simulink model "sampleModel1592"  (R2023a)
settings: Solver=VariableStepAuto  StartTime=0.0  StopTime=10.0  RelTol=1e-3
libraries: hdlsllib x2, simulink x1
settings Model: Creator=user1  LastModifiedBy=user1

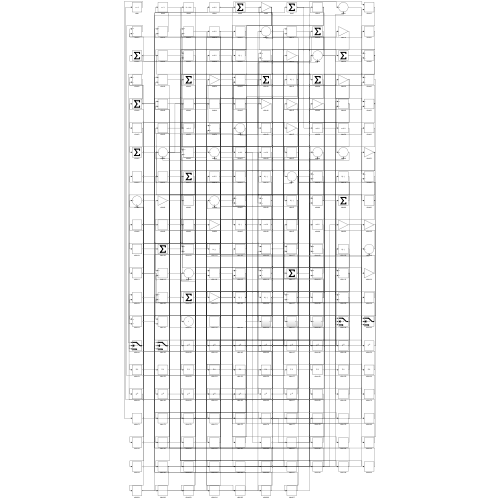
[thumbnail: Simulink's stored preview of the top-level diagram]
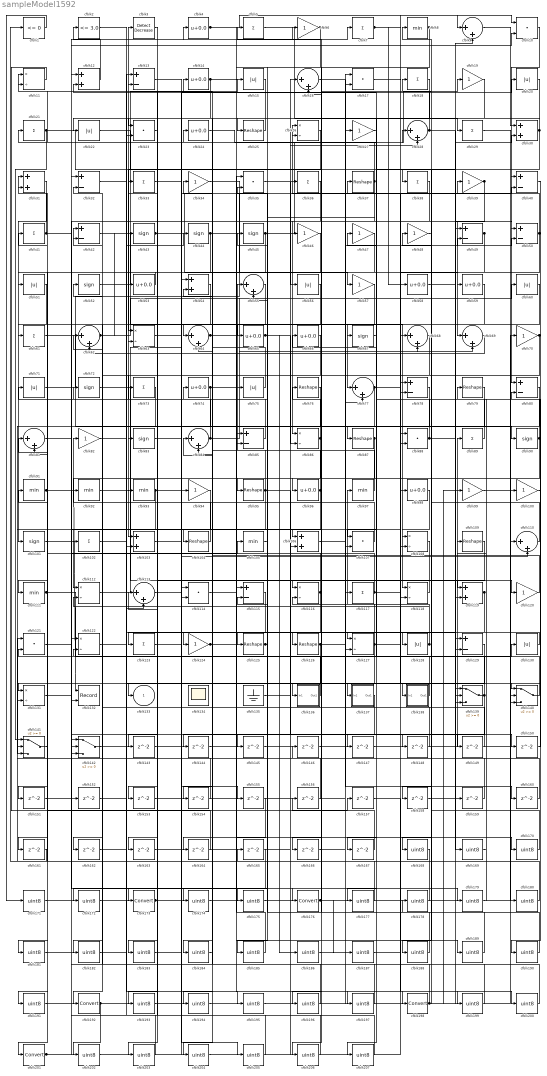
== system sampleModel1592 ==
  cfblk1 : hdlsllib/Logic and Bit Operations/Compare To Zero  relop=<=  OutDataTypeStr=boolean
  cfblk{10,17,23,35,88,107,114,121} (8 alike) : DotProduct  OutDataTypeStr=Inherit: Inherit via internal rule
  cfblk{6,19,27,34,39,46..48,57,70,82,94,99..100,120,124} (16 alike) : Gain
  cfblk{43..45,52,67,72,83,90,101} (9 alike) : Signum
  cfblk{5,7,18,21,29,33,36,38,41,61,73,89,102,117,123} (15 alike) : Sum  Inputs=+
  cfblk{12,30..31,54,103,106,119} (7 alike) : Sum
  cfblk{25,37,76,79,87,95,104,109,125..126} (10 alike) : Reshape
  cfblk{8,91..93,97,105,111} (7 alike) : MinMax
  cfblk{11,26,63,86,108,112,116,118,122,127,131} (11 alike) : Product  Inputs=*/  RndMeth=Zero  SaturateOnIntegerOverflow=on
  cfblk{9,16,28,55,62,64,68..69,77,81,84,110,113} (13 alike) : Sum  Inputs=|++
  cfblk{13,32,40,42,49..50,78,80,85,115,129} (11 alike) : Sum  Inputs=+-
  cfblk{15,20,22,51,56,60,71,75,128,130} (10 alike) : Abs  SaturateOnIntegerOverflow=off
  cfblk132 : Record  FileSettingsInternal="{\"entries\":[{\"content\":{\"excelSettings\":{\"content\":{},\"type\":\"Streamout.ExcelSettings\"}},\"type\":\"Streamout.FileSettingStorage\",\"uuid\":\"\"}],\"packageUris\":[\"http:\\/\\/schema.mathworks.com\\/mf0\\/streamout_blocks\\/R2020a\"],\"version\":\"1.0\"}"  Layout=[1 1]  SignalsInternal="{\"entries\":[{\"content\":{\"signals\":[{\"content\":{\"blockPath\":[],\"dimensions\":[1],\"domain\":\"\",\"lineColor\":\"#a2142f\",\"plots\":[1],\"port\":1,\"signalID\":2175,\"signalName\":\"XY Graph:1\"},\"type\":\"RecordBlkView.Signal\",\"uuid\":\"\"},{\"content\":{\"blockPath\":[],\"dimensions\":[1],\"domain\":\"\",\"lineColor\":\"#139fff\",\"plots\":[1],\"port\":2,\"signalID\":2178,\"signalName\":\"XY Graph:2\"},\"type\":\"RecordBlkView.Signal\",\"uuid\":\"\"}]},\"type\":\"RecordBlkView.InputSignals\",\"uuid\":\"\"}],\"packageUris\":[\"http:\\/\\/schema.mathworks.com\\/mf0\\/streamout_blocks\\/R2020a\"],\"version\":\"1.0\"}"  VisualizationBindings="{\"xyplotplugin\":{\"info\":[{\"series\":[{\"bindingParametersList\":[{\"parameter\":\"X-Axis\",\"signalID\":2175,\"signalName\":\"XY Graph:1\"},{\"parameter\":\"Y-Axis\",\"signalID\":2178,\"signalName\":\"XY Graph:2\"}],\"seriesID\":40184}],\"subplotID\":1}]}}"  CompatibilityTag=XY  st=-1
  cfblk134 : Scope
      settings: Floating=on
  cfblk135 : Ground
  cfblk136 : Subsystem
      settings: LibrarySourceBlock=|
      | hdlsllib/Ports &
      | Subsystems/Subsystem
  cfblk137 : Subsystem
      settings: LibrarySourceBlock=|
      | hdlsllib/Ports &
      | Subsystems/Subsystem
  cfblk138 : Subsystem
      settings: LibrarySourceBlock=|
      | hdlsllib/Ports &
      | Subsystems/Subsystem
  cfblk{139..142} (4 alike) : Switch  SaturateOnIntegerOverflow=off  InputSameDT=off
  cfblk{4,14,24,53,58..59,65..66,74,96,98} (11 alike) : Bias  Bias=0.0  SaturateOnIntegerOverflow=off
  cfblk{143..167} (25 alike) : Delay  SampleTime=1
  cfblk{168..172,174..175,177..191,193..197,199..200,202..207} (35 alike) : DataTypeConversion  OutDataTypeStr=uint8  SaturateOnIntegerOverflow=off  RndMeth=Floor
  cfblk{173,176,192,198,201} (5 alike) : DataTypeConversion  SaturateOnIntegerOverflow=off  RndMeth=Floor
  cfblk2 : hdlsllib/Logic and Bit Operations/Compare To Constant  relop=<=  const=3.0  OutDataTypeStr=boolean
  cfblk3 : simulink/Logic and Bit Operations/Detect Decrease  vinit=0.0  OutDataTypeStr=boolean
      settings: LibrarySourceBlock=|
      | hdlsllib/Logic and Bit
      | Operations/Detect
      | Decrease
  cfblk133 : Outport  VectorParamsAs1DForOutWhenUnconnected=off
  wires:
  cfblk20/1 -> cfblk80/1
  cfblk40/1 -> cfblk140/1
  cfblk4/1 -> cfblk9/1, cfblk38/1
  cfblk38/1 -> cfblk86/1
  cfblk52/1 -> cfblk15/1
  cfblk71/1 -> cfblk37/1
  cfblk32/1 -> cfblk198/1
  cfblk130/1 -> cfblk123/1
  cfblk116/1 -> cfblk125/1, cfblk91/1
  cfblk6/1 -> cfblk25/1, cfblk85/2, cfblk175/1
  cfblk24/1 -> cfblk19/1
  cfblk115/1 -> cfblk173/1
  cfblk37/1 -> cfblk64/1, cfblk142/3, cfblk11/2
  cfblk31/1 -> cfblk101/1
  cfblk111/1 -> cfblk130/1, cfblk105/1
  cfblk75/1 -> cfblk24/1
  cfblk61/1 -> cfblk87/1
  cfblk97/1 -> cfblk55/1
  cfblk62/1 -> cfblk60/1, cfblk44/1, cfblk43/1
  cfblk45/1 -> cfblk28/1, cfblk64/2
  cfblk85/1 -> cfblk3/1
  cfblk26/1 -> cfblk63/1
  cfblk39/1 -> cfblk69/1, cfblk194/1
  cfblk136/1(Out1) -> cfblk81/1
  cfblk110/1 -> cfblk8/1
  cfblk142/1 -> cfblk89/1
  cfblk8/1 -> cfblk136/1(In1), cfblk16/2
  cfblk124/1 -> cfblk126/1, cfblk189/1
  cfblk64/1 -> cfblk124/1, cfblk67/1
  cfblk60/1 -> cfblk111/1
  cfblk117/1 -> cfblk33/1, cfblk50/2
  cfblk104/1 -> cfblk82/1
  cfblk92/1 -> cfblk120/1
  cfblk91/1 -> cfblk132/1, cfblk10/2
  cfblk128/1 -> cfblk97/1, cfblk112/2
  cfblk53/1 -> cfblk51/1
  cfblk10/1 -> cfblk40/1
  cfblk47/1 -> cfblk96/1
  cfblk15/1 -> cfblk104/1
  cfblk112/1 -> cfblk20/1
  cfblk66/1 -> cfblk103/1
  cfblk80/1 -> cfblk84/2
  cfblk88/1 -> cfblk129/1, cfblk66/1
  cfblk42/1 -> cfblk118/1
  cfblk103/1 -> cfblk39/1
  cfblk96/1 -> cfblk133/1, cfblk11/1
  cfblk9/1 -> cfblk30/1
  cfblk74/1 -> cfblk69/2, cfblk141/3
  cfblk46/1 -> cfblk95/1
  cfblk67/1 -> cfblk137/1(In1)
  cfblk30/1 -> cfblk128/1, cfblk22/1, cfblk167/1
  cfblk78/1 -> cfblk192/1
  cfblk5/1 -> cfblk29/1
  cfblk139/1 -> cfblk74/1, cfblk166/1
  cfblk50/1 -> cfblk26/1, cfblk131/1
  cfblk107/1 -> cfblk42/1
  cfblk43/1 -> cfblk26/2, cfblk57/1
  cfblk18/1 -> cfblk127/1
  cfblk127/1 -> cfblk6/1, cfblk40/2, cfblk132/2
  cfblk81/1 -> cfblk4/1
  cfblk35/1 -> cfblk56/1
  cfblk12/1 -> cfblk2/1
  cfblk98/1 -> cfblk108/1
  cfblk126/1 -> cfblk27/1, cfblk181/1
  cfblk93/1 -> cfblk138/1(In1), cfblk161/1
  cfblk28/1 -> cfblk5/1, cfblk50/1, cfblk30/2
  cfblk2/1 -> cfblk129/2
  cfblk84/1 -> cfblk46/1, cfblk71/1, cfblk62/1
  cfblk86/1 -> cfblk76/1, cfblk144/1
  cfblk21/1 -> cfblk141/1, cfblk139/2
  cfblk22/1 -> cfblk88/1
  cfblk14/1 -> cfblk103/2, cfblk200/1
  cfblk89/1 -> cfblk12/2
  cfblk41/1 -> cfblk31/1, cfblk7/1, cfblk108/2
  cfblk72/1 -> cfblk106/1
  cfblk95/1 -> cfblk131/2, cfblk62/2, cfblk148/1
  cfblk94/1 -> cfblk201/1
  cfblk59/1 -> cfblk77/1
  cfblk118/1 -> cfblk116/1
  cfblk51/1 -> cfblk61/1
  cfblk87/1 -> cfblk93/1, cfblk162/1
  cfblk3/1 -> cfblk83/1
  cfblk120/1 -> cfblk14/1
  cfblk90/1 -> cfblk21/1, cfblk196/1
  cfblk65/1 -> cfblk90/1, cfblk186/1
  cfblk7/1 -> cfblk10/1, cfblk119/1, cfblk58/1
  cfblk140/1 -> cfblk47/1
  cfblk82/1 -> cfblk140/2
  cfblk69/1 -> cfblk63/2
  cfblk105/1 -> cfblk75/1
  cfblk138/1(Out1) -> cfblk52/1
  cfblk55/1 -> cfblk65/1
  cfblk25/1 -> cfblk23/1
  cfblk17/1 -> cfblk59/1
  cfblk44/1 -> cfblk16/1, cfblk53/1, cfblk174/1
  cfblk99/1 -> cfblk140/3
  cfblk34/1 -> cfblk117/1
  cfblk49/1 -> cfblk107/1, cfblk207/1
  cfblk121/1 -> cfblk176/1
  cfblk135/1 -> cfblk28/2
  cfblk77/1 -> cfblk86/2, cfblk102/1, cfblk139/3
  cfblk125/1 -> cfblk85/1, cfblk45/1
  cfblk119/1 -> cfblk153/1, cfblk154/1
  cfblk141/1 -> cfblk41/1
  cfblk83/1 -> cfblk110/2
  cfblk106/1 -> cfblk49/2
  cfblk101/1 -> cfblk112/1
  cfblk70/1 -> cfblk92/1, cfblk158/1
  cfblk102/1 -> cfblk73/1
  cfblk56/1 -> cfblk143/1
  cfblk143/1 -> cfblk9/2
  cfblk144/1 -> cfblk118/2
  cfblk76/1 -> cfblk145/1
  cfblk145/1 -> cfblk127/2
  cfblk146/1 -> cfblk17/2
  cfblk63/1 -> cfblk147/1
  cfblk147/1 -> cfblk110/1
  cfblk148/1 -> cfblk42/2
  cfblk131/1 -> cfblk149/1
  cfblk149/1 -> cfblk84/1
  cfblk123/1 -> cfblk150/1
  cfblk150/1 -> cfblk80/2
  cfblk129/1 -> cfblk151/1
  cfblk151/1 -> cfblk12/1
  cfblk152/1 -> cfblk23/2
  cfblk153/1 -> cfblk107/2
  cfblk154/1 -> cfblk31/2
  cfblk33/1 -> cfblk155/1
  cfblk156/1 -> cfblk55/2
  cfblk11/1 -> cfblk157/1
  cfblk158/1 -> cfblk139/1
  cfblk159/1 -> cfblk141/2
  cfblk16/1 -> cfblk160/1
  cfblk160/1 -> cfblk49/1
  cfblk161/1 -> cfblk1/1
  cfblk109/1 -> cfblk163/1
  cfblk163/1 -> cfblk106/2
  cfblk137/1(Out1) -> cfblk164/1
  cfblk164/1 -> cfblk81/2
  cfblk166/1 -> cfblk77/2
  cfblk167/1 -> cfblk116/2
  cfblk79/1 -> cfblk168/1
  cfblk168/1 -> cfblk165/1
  cfblk58/1 -> cfblk169/1
  cfblk169/1 -> cfblk79/1
  cfblk114/1 -> cfblk170/1
  cfblk170/1 -> cfblk18/1
  cfblk1/1 -> cfblk171/1
  cfblk171/1 -> cfblk114/1
  cfblk165/1 -> cfblk172/1
  cfblk172/1 -> cfblk114/2
  cfblk173/1 -> cfblk159/1, cfblk70/1
  cfblk174/1 -> cfblk115/1
  cfblk175/1 -> cfblk115/2
  cfblk176/1 -> cfblk156/1, cfblk88/2, cfblk187/1
  cfblk27/1 -> cfblk177/1
  cfblk177/1 -> cfblk121/1
  cfblk178/1 -> cfblk121/2
  cfblk113/1 -> cfblk179/1
  cfblk179/1 -> cfblk109/1
  cfblk29/1 -> cfblk180/1
  cfblk180/1 -> cfblk113/1
  cfblk181/1 -> cfblk113/2
  cfblk54/1 -> cfblk182/1
  cfblk182/1 -> cfblk72/1
  cfblk23/1 -> cfblk183/1
  cfblk183/1 -> cfblk54/1
  cfblk155/1 -> cfblk184/1
  cfblk184/1 -> cfblk54/2
  cfblk68/1 -> cfblk185/1
  cfblk185/1 -> cfblk35/1
  cfblk186/1 -> cfblk68/1
  cfblk187/1 -> cfblk68/2
  cfblk48/1 -> cfblk188/1
  cfblk188/1 -> cfblk35/2
  cfblk189/1 -> cfblk48/1
  cfblk100/1 -> cfblk190/1
  cfblk190/1 -> cfblk146/1
  cfblk73/1 -> cfblk191/1
  cfblk191/1 -> cfblk100/1
  cfblk192/1 -> cfblk119/2, cfblk202/1
  cfblk57/1 -> cfblk193/1
  cfblk193/1 -> cfblk78/1
  cfblk194/1 -> cfblk78/2
  cfblk122/1 -> cfblk195/1
  cfblk195/1 -> cfblk17/1
  cfblk196/1 -> cfblk122/1
  cfblk162/1 -> cfblk197/1
  cfblk197/1 -> cfblk122/2
  cfblk198/1 -> cfblk178/1, cfblk99/1, cfblk34/1
  cfblk157/1 -> cfblk199/1
  cfblk199/1 -> cfblk32/1
  cfblk200/1 -> cfblk32/2
  cfblk201/1 -> cfblk152/1, cfblk98/1
  cfblk202/1 -> cfblk94/1
  cfblk36/1 -> cfblk203/1
  cfblk203/1 -> cfblk142/1
  cfblk108/1 -> cfblk204/1
  cfblk204/1 -> cfblk36/1
  cfblk13/1 -> cfblk205/1
  cfblk205/1 -> cfblk142/2
  cfblk19/1 -> cfblk206/1
  cfblk206/1 -> cfblk13/1
  cfblk207/1 -> cfblk13/2

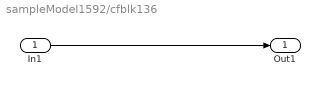
== system sampleModel1592/cfblk136 ==
  In1 : Inport
  Out1 : Outport
  wires:
  In1/1 -> Out1/1

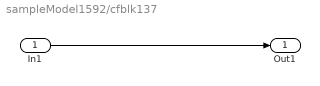
== system sampleModel1592/cfblk137 ==
  In1 : Inport
  Out1 : Outport
  wires:
  In1/1 -> Out1/1

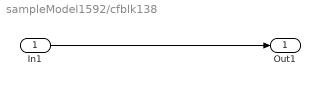
== system sampleModel1592/cfblk138 ==
  In1 : Inport
  Out1 : Outport
  wires:
  In1/1 -> Out1/1
